simulink model "simu1"  (R2024a)
settings: Solver=VariableStepAuto  StartTime=0.0  StopTime=10.0  RelTol=1e-3
settings Model: Creator=psp_dada  LastModifiedBy=psp_dada

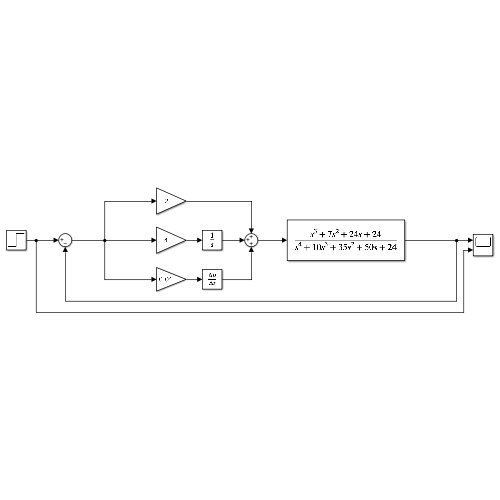
[thumbnail: Simulink's stored preview of the top-level diagram]
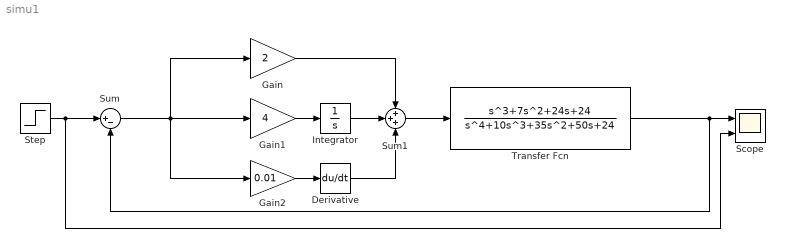
== system simu1 ==
  Derivative : Derivative
  Gain : Gain  Gain=2
  Gain1 : Gain  Gain=4
  Gain2 : Gain  Gain=0.01
  Integrator : Integrator
  Scope : Scope  NumInputPorts=2
  Step : Step  SampleTime=0.01
  Sum : Sum  Inputs=|+-
  Sum1 : Sum  Inputs=+++
  Transfer Fcn : TransferFcn  Numerator=[1 7 24 24]  Denominator=[1 10 35 50 24]
  wires:
  Step/1 -> Scope/2, Sum/1
  Sum/1 -> Gain/1, Gain2/1, Gain1/1
  Gain2/1 -> Derivative/1
  Gain1/1 -> Integrator/1
  Transfer Fcn/1 -> Sum/2, Scope/1
  Integrator/1 -> Sum1/2
  Derivative/1 -> Sum1/3
  Gain/1 -> Sum1/1
  Sum1/1 -> Transfer Fcn/1
